simulink model "ST_ESP_ESM_2016a"  (R2016a)
settings: Solver=ode1  StartTime=0.0  StopTime=SIM_time  FixedStep=stepsize  RelTol=1e-3
values from neighbouring files (symbols this model uses):
  A = 2.26    [ST_einspur_parameter.m]
  brems_k_max = 25000    [ST_einspur_parameter.m]
  cw = 0.32    [ST_einspur_parameter.m]
  delta_lr = 0    [ST_einspur_parameter_dynamik.m]    (also in ST_einspur_parameter_sinus.m = 90; ST_einspur_parameter_sprung.m = 90)
  fah_dkv = 0.6    [ST_einspur_parameter_dynamik.m]    (also in ST_einspur_parameter_sinus.m = 0.2; ST_einspur_parameter_sprung.m)
  fzg_Jz = 3489    [ST_einspur_parameter.m]
  fzg_l = 2.758    [ST_einspur_parameter.m]
  fzg_lh = fzg_l-fzg_lv    (= 1.158)    [ST_einspur_parameter.m]
  fzg_lv = 1.6    [ST_einspur_parameter.m]
  fzg_m = 1700    [ST_einspur_parameter.m]
  fzg_s = 1.7    [ST_einspur_parameter.m]
  g = 9.81    [ST_einspur_parameter.m]
  h_sp = 0.56    [ST_einspur_parameter.m]
  i_diff = 3.5    [ST_einspur_parameter.m]
  i_getr = 4.2    [ST_einspur_parameter.m]
  i_lenk = 18    [ST_einspur_parameter.m]
  init_v0 = 5/3.6    (= 1.38888888889)    [ST_einspur_parameter_dynamik.m]    (also in ST_einspur_parameter_sinus.m = 13.8888888889; ST_einspur_parameter_sprung.m = 11.1111111111)
  len_wahl = 1    [ST_einspur_parameter_dynamik.m]    (also in ST_einspur_parameter_sinus.m = 2; ST_einspur_parameter_sprung.m = 3)
  mue_h = 1.0    (= 1)    [ST_einspur_parameter.m]
  mue_v = 1.0    (= 1)    [ST_einspur_parameter.m]
  omega_max = 630    [ST_einspur_parameter.m]
  p_max = 110000    [ST_einspur_parameter.m]
  rad_r = 0.31    [ST_einspur_parameter.m]
  rho = 1.226    [ST_einspur_parameter.m]
  sin_freq = pi/2    (= 1.57079632679)    [ST_einspur_parameter_dynamik.m]    (also in ST_einspur_parameter_sinus.m = 1.0471975512; ST_einspur_parameter_sprung.m)
  step_time = 1    [ST_einspur_parameter_dynamik.m]    (also in ST_einspur_parameter_sinus.m; ST_einspur_parameter_sprung.m = 3)
  sw_ESP = 1    [ST_einspur_parameter_sinus.m]    (also in ST_einspur_parameter_sprung.m)
libraries: simulink x2
(part 1 of 2)
settings Model: Creator=os.alsaidi  LastModifiedBy=Yuheng_Wu
settings DataIOCC: LimitDataPoints=on  SaveFormat=Array
settings HardwareCC: ProdBitPerPointer=32  ProdLargestAtomicFloat=None  ProdIntDivRoundTo=Undefined  ProdEndianess=Unspecified  ProdWordSize=32  ProdHWDeviceType=32-bit Generic
settings ModelReferenceCC: PropagateSignalLabelsOutOfModel=off

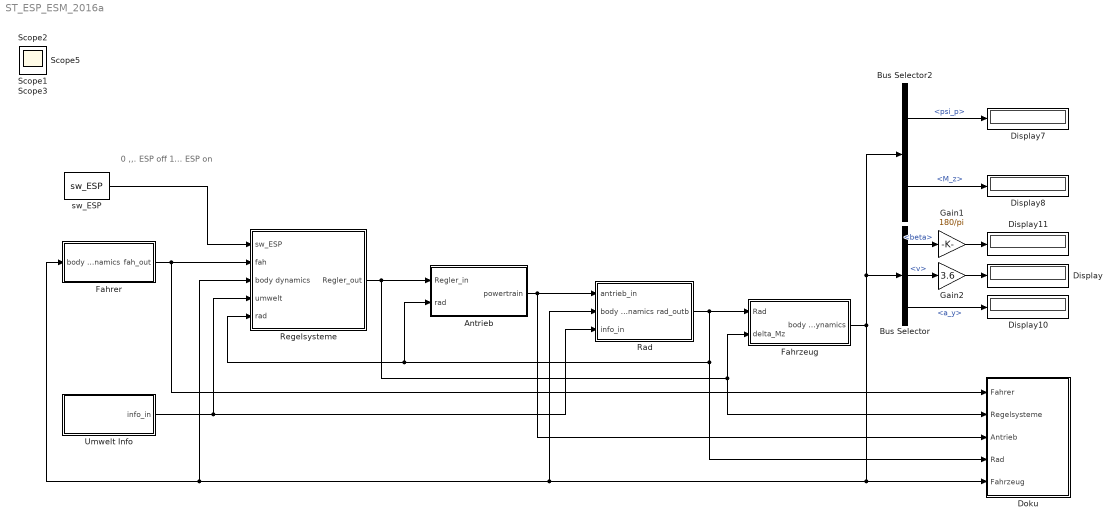
== system ST_ESP_ESM_2016a ==
  note: 0 ,,. ESP off
      | 1... ESP on
  Antrieb : Subsystem
  Bus Selector : BusSelector  OutputSignals=beta,v,a_y
  Bus Selector2 : BusSelector  OutputSignals=psi_p,M_z
  Display{,7..8,10..11} (5 alike) : Display
  Doku : Subsystem
  Fahrer : Subsystem
  Fahrzeug : Subsystem
  Gain1 : Gain  Gain=180/pi
  Gain2 : Gain  Gain=3.6
  Rad : Subsystem
      mask help: Simulink:masks:GenSFuncDesc_MD
      mask Help: eval('feval(''rtwprivate'',''rtwhelpview'',''rtw_sfcn_block'')');
  Regelsysteme : Subsystem
  Umwelt Info : Subsystem
  sw_ESP : Constant  Value=sw_ESP
  Scope{1..3,5} (4 alike) : Scope
  wires:
  Fahrzeug/1(body dynamics) -> Doku/5(Fahrzeug), Rad/2(body dynamics), Regelsysteme/3(body dynamics), Fahrer/1(body dynamics), Bus Selector/1, Bus Selector2/1
  Fahrer/1(fah_out) -> Doku/1(Fahrer), Regelsysteme/2(fah)
  Rad/1(rad_outb) -> Doku/4(Rad), Antrieb/2(rad), Regelsysteme/5(rad), Fahrzeug/1(Rad)
  Antrieb/1(powertrain) -> Rad/1(antrieb_in), Doku/3(Antrieb)
  Bus Selector/2 -> Gain2/1  "<v>"
  Umwelt Info/1(info_in) -> Rad/3(info_in), Regelsysteme/4(umwelt)
  Regelsysteme/1(Regler_out) -> Antrieb/1(Regler_in), Fahrzeug/2(delta_Mz), Doku/2(Regelsysteme)
  Bus Selector/3 -> Display10/1  "<a_y>"
  Bus Selector/1 -> Gain1/1  "<beta>"
  Gain1/1 -> Display11/1
  Gain2/1 -> Display/1
  Bus Selector2/1 -> Display7/1  "<psi_p>"
  Bus Selector2/2 -> Display8/1  "<M_z>"
  sw_ESP/1 -> Regelsysteme/1(sw_ESP)

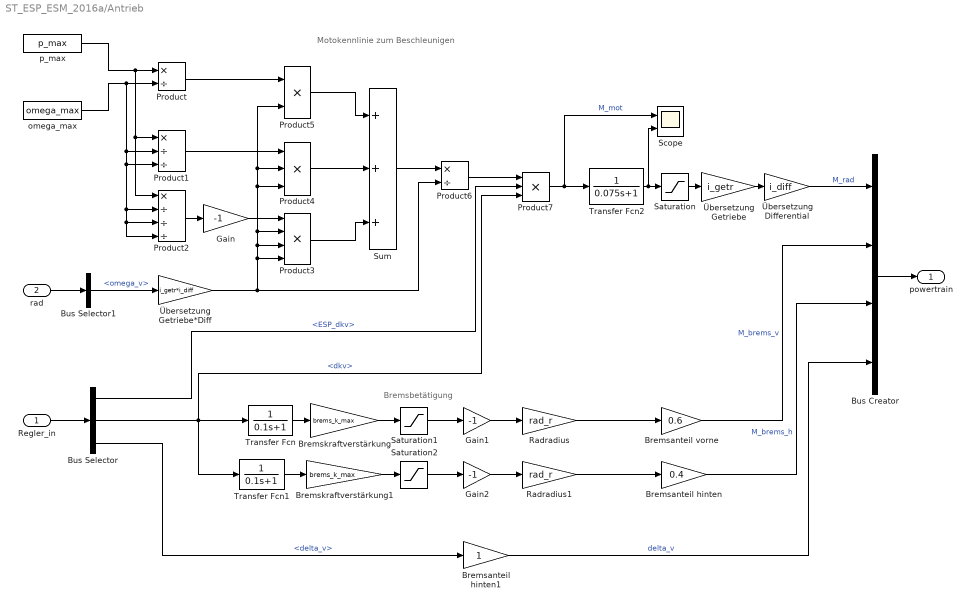
== system ST_ESP_ESM_2016a/Antrieb ==
  note: Motokennlinie zum Beschleunigen
  note: Bremsbetätigung
  Regler_in : Inport
  rad : Inport  Port=2
  Bremsanteil hinten : Gain  Gain=0.4
  Bremsanteil hinten1 : Gain
  Bremsanteil vorne : Gain  Gain=0.6
  Bremskraftverstärkung : Gain  Gain=brems_k_max
  Bremskraftverstärkung1 : Gain  Gain=brems_k_max
  Bus Creator : BusCreator  Inputs=4
  Bus Selector : BusSelector  OutputSignals=ESP.ESP_dkv,fahrer.dkv,fahrer.delta_v
  Bus Selector1 : BusSelector  OutputSignals=omega_v
  Gain : Gain  Gain=-1
  Gain1 : Gain  Gain=-1
  Gain2 : Gain  Gain=-1
  Product : Product  Inputs=*/  RndMeth=Zero
  Product1 : Product  Inputs=*//  RndMeth=Zero
  Product2 : Product  Inputs=*///  RndMeth=Zero
  Product3 : Product  Inputs=4  RndMeth=Zero
  Product4 : Product  Inputs=3  RndMeth=Zero
  Product5 : Product  RndMeth=Zero
  Product6 : Product  Inputs=*/  RndMeth=Zero
  Product7 : Product  Inputs=3  RndMeth=Zero
  Radradius : Gain  Gain=rad_r
  Radradius1 : Gain  Gain=rad_r
  Saturation : Saturate  UpperLimit=inf  LowerLimit=0
  Saturation1 : Saturate  UpperLimit=0  LowerLimit=-inf
  Saturation2 : Saturate  UpperLimit=0  LowerLimit=-inf
  Scope : Scope  NumInputPorts=2
  Sum : Sum  Inputs=+++
  Transfer Fcn : TransferFcn  Denominator=[0.1 1]
  Transfer Fcn1 : TransferFcn  Denominator=[0.1 1]
  Transfer Fcn2 : TransferFcn  Denominator=[0.075 1]
  omega_max : Constant  Value=omega_max
  p_max : Constant  Value=p_max
  Übersetzung Differential : Gain  Gain=i_diff
  Übersetzung Getriebe : Gain  Gain=i_getr
  Übersetzung Getriebe*Diff : Gain  Gain=i_getr*i_diff
  powertrain : Outport
  wires:
  rad/1 -> Bus Selector1/1
  Bus Selector1/1 -> Übersetzung Getriebe*Diff/1  "<omega_v>"
  p_max/1 -> Product/1, Product1/1, Product2/1
  omega_max/1 -> Product/2, Product1/2, Product1/3, Product2/2, Product2/3, Product2/4
  Product/1 -> Product5/1
  Product2/1 -> Gain/1
  Product1/1 -> Product4/1
  Gain/1 -> Product3/1
  Product5/1 -> Sum/1
  Product4/1 -> Sum/2
  Product3/1 -> Sum/3
  Sum/1 -> Product6/1
  Product6/1 -> Product7/1
  Product7/1 -> Scope/1, Transfer Fcn2/1  "M_mot"
  Übersetzung Getriebe/1 -> Übersetzung Differential/1
  Übersetzung Differential/1 -> Bus Creator/1  "M_rad"
  Bus Creator/1 -> powertrain/1
  Saturation/1 -> Übersetzung Getriebe/1
  Bremskraftverstärkung/1 -> Saturation1/1
  Saturation1/1 -> Gain1/1
  Gain1/1 -> Radradius/1
  Bremsanteil vorne/1 -> Bus Creator/2  "M_brems_v"
  Radradius/1 -> Bremsanteil vorne/1
  Bremsanteil hinten/1 -> Bus Creator/3  "M_brems_h"
  Bremskraftverstärkung1/1 -> Saturation2/1
  Saturation2/1 -> Gain2/1
  Gain2/1 -> Radradius1/1
  Radradius1/1 -> Bremsanteil hinten/1
  Regler_in/1 -> Bus Selector/1
  Bus Selector/3 -> Bremsanteil hinten1/1  "<delta_v>"
  Bus Selector/2 -> Product7/3, Transfer Fcn/1, Transfer Fcn1/1  "<dkv>"
  Übersetzung Getriebe*Diff/1 -> Product3/3, Product3/2, Product4/3, Product4/2, Product5/2, Product3/4, Product6/2
  Transfer Fcn/1 -> Bremskraftverstärkung/1
  Transfer Fcn1/1 -> Bremskraftverstärkung1/1
  Transfer Fcn2/1 -> Scope/2, Saturation/1
  Bremsanteil hinten1/1 -> Bus Creator/4  "delta_v"
  Bus Selector/1 -> Product7/2  "<ESP_dkv>"

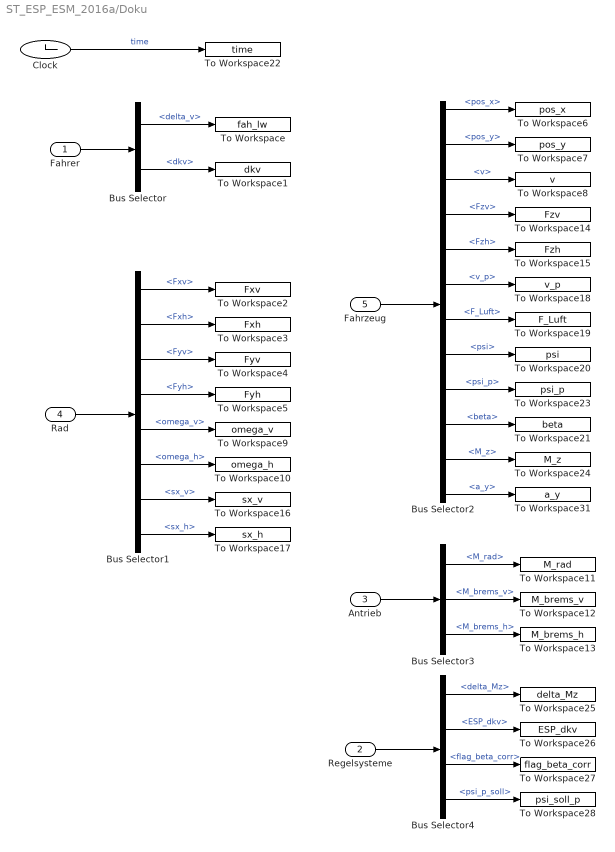
== system ST_ESP_ESM_2016a/Doku ==
  Fahrer : Inport
  Regelsysteme : Inport  Port=2
  Antrieb : Inport  Port=3
  Rad : Inport  Port=4
  Fahrzeug : Inport  Port=5
  Bus Selector : BusSelector  OutputSignals=delta_v,dkv
  Bus Selector1 : BusSelector  OutputSignals=Fxv,Fxh,Fyv,Fyh,omega_v,omega_h,sx_v,sx_h
  Bus Selector2 : BusSelector  OutputSignals=pos_x,pos_y,v,Fzv,Fzh,v_p,F_Luft,psi,psi_p,beta,M_z,a_y
  Bus Selector3 : BusSelector  OutputSignals=M_rad,M_brems_v,M_brems_h
  Bus Selector4 : BusSelector  OutputSignals=ESP.delta_Mz,ESP.ESP_dkv,ESP.flag_beta_corr,ESP.psi_p_soll
  Clock : Clock
  To Workspace : ToWorkspace  VariableName=fah_lw  SampleTime=-1
  To Workspace1 : ToWorkspace  VariableName=dkv  SampleTime=-1
  To Workspace10 : ToWorkspace  VariableName=omega_h  SampleTime=-1
  To Workspace11 : ToWorkspace  VariableName=M_rad  SampleTime=-1
  To Workspace12 : ToWorkspace  VariableName=M_brems_v  SampleTime=-1
  To Workspace13 : ToWorkspace  VariableName=M_brems_h  SampleTime=-1
  To Workspace14 : ToWorkspace  VariableName=Fzv  SampleTime=-1
  To Workspace15 : ToWorkspace  VariableName=Fzh  SampleTime=-1
  To Workspace16 : ToWorkspace  VariableName=sx_v  SampleTime=-1
  To Workspace17 : ToWorkspace  VariableName=sx_h  SampleTime=-1
  To Workspace18 : ToWorkspace  VariableName=v_p  SampleTime=-1
  To Workspace19 : ToWorkspace  VariableName=F_Luft  SampleTime=-1
  To Workspace2 : ToWorkspace  VariableName=Fxv  SampleTime=-1
  To Workspace20 : ToWorkspace  VariableName=psi  SampleTime=-1
  To Workspace21 : ToWorkspace  VariableName=beta  SampleTime=-1
  To Workspace22 : ToWorkspace  VariableName=time  SampleTime=-1
  To Workspace23 : ToWorkspace  VariableName=psi_p  SampleTime=-1
  To Workspace24 : ToWorkspace  VariableName=M_z  SampleTime=-1
  To Workspace25 : ToWorkspace  VariableName=delta_Mz  SampleTime=-1
  To Workspace26 : ToWorkspace  VariableName=ESP_dkv  SampleTime=-1
  To Workspace27 : ToWorkspace  VariableName=flag_beta_corr  SampleTime=-1
  To Workspace28 : ToWorkspace  VariableName=psi_soll_p  SampleTime=-1
      settings: Save2DSignal=2-D array (concatenate along first dimension)
  To Workspace3 : ToWorkspace  VariableName=Fxh  SampleTime=-1
  To Workspace31 : ToWorkspace  VariableName=a_y  SampleTime=-1
  To Workspace4 : ToWorkspace  VariableName=Fyv  SampleTime=-1
  To Workspace5 : ToWorkspace  VariableName=Fyh  SampleTime=-1
  To Workspace6 : ToWorkspace  VariableName=pos_x  SampleTime=-1
  To Workspace7 : ToWorkspace  VariableName=pos_y  SampleTime=-1
  To Workspace8 : ToWorkspace  VariableName=v  SampleTime=-1
  To Workspace9 : ToWorkspace  VariableName=omega_v  SampleTime=-1
  wires:
  Fahrer/1 -> Bus Selector/1
  Rad/1 -> Bus Selector1/1
  Fahrzeug/1 -> Bus Selector2/1
  Bus Selector/1 -> To Workspace/1  "<delta_v>"
  Bus Selector/2 -> To Workspace1/1  "<dkv>"
  Bus Selector1/1 -> To Workspace2/1  "<Fxv>"
  Bus Selector1/2 -> To Workspace3/1  "<Fxh>"
  Bus Selector1/3 -> To Workspace4/1  "<Fyv>"
  Bus Selector1/4 -> To Workspace5/1  "<Fyh>"
  Bus Selector2/1 -> To Workspace6/1  "<pos_x>"
  Bus Selector2/2 -> To Workspace7/1  "<pos_y>"
  Bus Selector2/3 -> To Workspace8/1  "<v>"
  Regelsysteme/1 -> Bus Selector4/1
  Bus Selector1/5 -> To Workspace9/1  "<omega_v>"
  Bus Selector1/6 -> To Workspace10/1  "<omega_h>"
  Antrieb/1 -> Bus Selector3/1
  Bus Selector3/1 -> To Workspace11/1  "<M_rad>"
  Bus Selector3/2 -> To Workspace12/1  "<M_brems_v>"
  Bus Selector3/3 -> To Workspace13/1  "<M_brems_h>"
  Bus Selector2/4 -> To Workspace14/1  "<Fzv>"
  Bus Selector2/5 -> To Workspace15/1  "<Fzh>"
  Bus Selector1/7 -> To Workspace16/1  "<sx_v>"
  Bus Selector1/8 -> To Workspace17/1  "<sx_h>"
  Bus Selector2/6 -> To Workspace18/1  "<v_p>"
  Bus Selector2/7 -> To Workspace19/1  "<F_Luft>"
  Bus Selector2/8 -> To Workspace20/1  "<psi>"
  Bus Selector2/10 -> To Workspace21/1  "<beta>"
  Clock/1 -> To Workspace22/1  "time"
  Bus Selector2/9 -> To Workspace23/1  "<psi_p>"
  Bus Selector2/11 -> To Workspace24/1  "<M_z>"
  Bus Selector4/1 -> To Workspace25/1  "<delta_Mz>"
  Bus Selector2/12 -> To Workspace31/1  "<a_y>"
  Bus Selector4/2 -> To Workspace26/1  "<ESP_dkv>"
  Bus Selector4/3 -> To Workspace27/1  "<flag_beta_corr>"
  Bus Selector4/4 -> To Workspace28/1  "<psi_p_soll>"

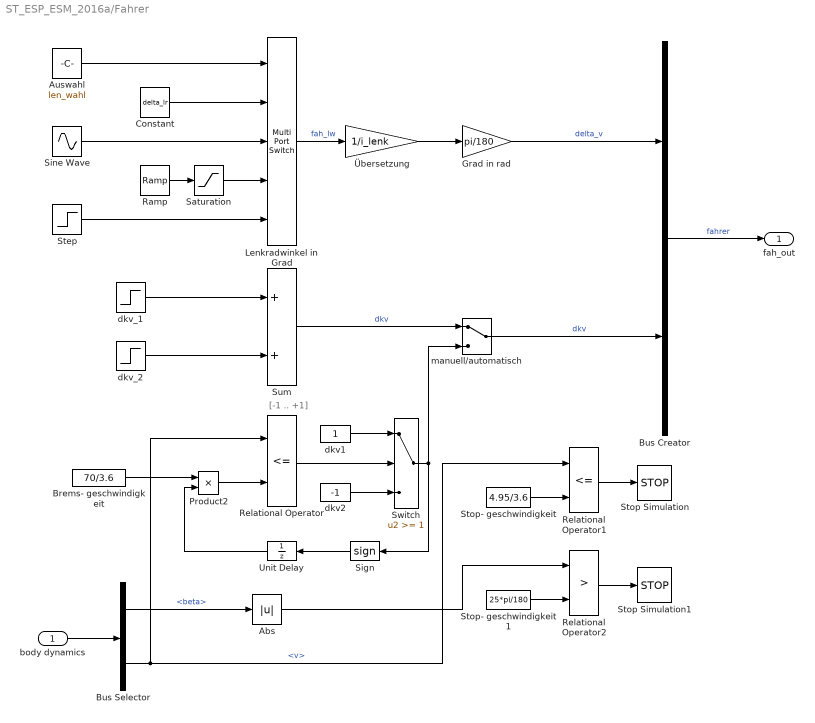
== system ST_ESP_ESM_2016a/Fahrer ==
  note: [-1 .. +1]
  body dynamics : Inport
  Abs : Abs
  Auswahl : Constant  Value=len_wahl
  Brems- geschwindigkeit : Constant  Value=70/3.6
  Bus Creator : BusCreator  Inputs=2
  Bus Selector : BusSelector  OutputSignals=beta,v
  Constant : Constant  Value=delta_lr
  Grad in rad : Gain  Gain=pi/180
  Lenkradwinkel in Grad : MultiPortSwitch  Inputs=4
  Product2 : Product  RndMeth=Zero
  Ramp : simulink/Sources/Ramp  slope=180/pi  start=step_time  X0=0
  Relational Operator : RelationalOperator  Operator=<=  OutDataTypeStr=boolean
  Relational Operator1 : RelationalOperator  Operator=<=  OutDataTypeStr=boolean
  Relational Operator2 : RelationalOperator  Operator=>  OutDataTypeStr=boolean
  Saturation : Saturate  UpperLimit=delta_lr  LowerLimit=-delta_lr
  Sign : Signum
  Sine Wave : Sin  Amplitude=delta_lr  Frequency=sin_freq  SampleTime=0
  Step : Step  Time=step_time+3  After=delta_lr  SampleTime=0
  Stop Simulation : Stop
  Stop Simulation1 : Stop
  Stop- geschwindigkeit : Constant  Value=4.95/3.6
  Stop- geschwindigkeit1 : Constant  Value=25*pi/180
  Sum : Sum
  Switch : Switch  Threshold=1
  Unit Delay : UnitDelay  InitialCondition=1  SampleTime=-1
  dkv1 : Constant
  dkv2 : Constant  Value=-1
  dkv_1 : Step  Time=0  Before=fah_dkv  After=fah_dkv  SampleTime=0
  dkv_2 : Step  Time=0  After=0  SampleTime=0
  manuell/automatisch : ManualSwitch
  Übersetzung : Gain  Gain=1/i_lenk
  fah_out : Outport
  wires:
  Auswahl/1 -> Lenkradwinkel in Grad/1
  Constant/1 -> Lenkradwinkel in Grad/2
  Sine Wave/1 -> Lenkradwinkel in Grad/3
  Ramp/1 -> Saturation/1
  Saturation/1 -> Lenkradwinkel in Grad/4
  dkv_1/1 -> Sum/1
  dkv_2/1 -> Sum/2
  Lenkradwinkel in Grad/1 -> Übersetzung/1  "fah_lw"
  Bus Creator/1 -> fah_out/1  "fahrer"
  Grad in rad/1 -> Bus Creator/1  "delta_v"
  manuell/automatisch/1 -> Bus Creator/2  "dkv"
  Sum/1 -> manuell/automatisch/1  "dkv"
  Relational Operator/1 -> Switch/2
  Switch/1 -> manuell/automatisch/2, Sign/1
  dkv1/1 -> Switch/1
  dkv2/1 -> Switch/3
  Brems- geschwindigkeit/1 -> Product2/1
  Product2/1 -> Relational Operator/2
  Unit Delay/1 -> Product2/2
  Sign/1 -> Unit Delay/1
  Stop- geschwindigkeit/1 -> Relational Operator1/2
  Relational Operator1/1 -> Stop Simulation/1
  Step/1 -> Lenkradwinkel in Grad/5
  Stop- geschwindigkeit1/1 -> Relational Operator2/2
  Relational Operator2/1 -> Stop Simulation1/1
  Übersetzung/1 -> Grad in rad/1
  body dynamics/1 -> Bus Selector/1
  Bus Selector/2 -> Relational Operator/1, Relational Operator1/1  "<v>"
  Bus Selector/1 -> Abs/1  "<beta>"
  Abs/1 -> Relational Operator2/1

== system ST_ESP_ESM_2016a/Fahrzeug ==
  Rad : Inport
  delta_Mz : Inport  Port=2
  "Bewegungsgleichungen " : Subsystem
  Bus Creator : BusCreator  Inputs=18
  Bus Selector : BusSelector  OutputSignals=Fxv,Fxh,Fyv,Fyh,delta_v
  Bus Selector2 : BusSelector  OutputSignals=ESP.delta_Mz
  Memory : Memory  X0=fzg_m*g*fzg_lh/(fzg_lh+fzg_lv)
  Memory1 : Memory  X0=fzg_m*g*fzg_lv/(fzg_lh+fzg_lv)
  Radaufstandskräfte : Subsystem
  x-y-Koordinaten : Subsystem
  body dynamics : Outport
  wires:
  Bus Selector2/1 -> "Bewegungsgleichungen "/6(delta_Mz)  "<delta_Mz>"
  delta_Mz/1 -> Bus Selector2/1
  "Bewegungsgleichungen "/9(a_x) -> Radaufstandskräfte/1(a_x), Bus Creator/16  "a_x"
  "Bewegungsgleichungen "/1(psi) -> Bus Creator/8, x-y-Koordinaten/1(psi)
  "Bewegungsgleichungen "/3(v) -> Bus Creator/10, x-y-Koordinaten/3(v)
  x-y-Koordinaten/2(pos_y) -> Bus Creator/7  "pos_y"
  Bus Selector/1 -> Bus Creator/1, "Bewegungsgleichungen "/1(Fxv)  "<Fxv>"
  Bus Selector/2 -> Bus Creator/2, "Bewegungsgleichungen "/2(Fxh)  "<Fxh>"
  Bus Selector/3 -> Bus Creator/3, "Bewegungsgleichungen "/3(Fyv)  "<Fyv>"
  Bus Selector/4 -> Bus Creator/4, "Bewegungsgleichungen "/4(Fyh)  "<Fyh>"
  Bus Selector/5 -> Bus Creator/5, "Bewegungsgleichungen "/5(delta_v)  "<delta_v>"
  Rad/1 -> Bus Selector/1
  Bus Creator/1 -> body dynamics/1
  x-y-Koordinaten/1(pos_x) -> Bus Creator/6  "pos_x"
  "Bewegungsgleichungen "/5(F_Luft) -> Radaufstandskräfte/2(F_luft), Bus Creator/12
  "Bewegungsgleichungen "/6(psi_p) -> Bus Creator/13
  Memory1/1 -> Bus Creator/18  "Fzh"
  Memory/1 -> Bus Creator/17  "Fzv"
  "Bewegungsgleichungen "/7(a_y) -> Bus Creator/14  "a_y"
  "Bewegungsgleichungen "/8(M_z) -> Bus Creator/15  "M_z"
  "Bewegungsgleichungen "/2(beta) -> Bus Creator/9, x-y-Koordinaten/2(beta)
  Radaufstandskräfte/1(Fzv) -> Memory/1
  Radaufstandskräfte/2(Fzh) -> Memory1/1
  "Bewegungsgleichungen "/4(v_p) -> Bus Creator/11  "v_p"

== system ST_ESP_ESM_2016a/Rad ==
  antrieb_in : Inport
  body dynamics : Inport  Port=2
  info_in : Inport  Port=3
  Rad_sfcn : S-Function  FunctionName=Rad_sf  SFunctionModules=""  SFunctionDeploymentMode=off  EnableBusSupport=off  mask{rtw_sf_name=Rad_sf, showVar=off}
      mask prompts: rtw_sf_name "Simulink:masks:GenSFuncName_MP"; showVar "Simulink:masks:GenSFuncShowModuleList_MP"
      mask help: Simulink:masks:GenSFuncDesc_MD
      mask init:
      | displist = '';
      | if ~strcmp(get_param(gcb, 'FunctionName'), rtw_sf_name);
      |   set_param(gcb, 'FunctionName', rtw_sf_name);
      | end
      | % Check if we are generating code
      | rtw_mode = false;
      | if strcmpi(get_param(bdroot(gcb),'SimulationStatus'),'Initializing')
      | 	rtw_mode = strcmpi(get_param(bdroot(gcb),'BuildingRTWCode'),'on') && ...
      | 		~strcmpi(get_param(bdroot(gcb),'TargetStyle'),'SimulationTarget');
      | end
      | if showVar || rtw_mode
      | 	if exist('rtwsfunc') == 2 | exist('rtwsfunc') == 6
      | 		tmplist = rtwsfunc(rtw_sf_name,gcb);
      | 		tmplist = DAStudio.message('Simulink:masks:GenSFuncListOfModules_IC', tmplist);
      | 	elseif showVar
      | 		tmplist1 = DAStudio.message('Simulink:masks:GenSFuncListOfModules_IC', '');
      |         tmplist2 = DAStudio.message('Simulink:masks:GenSFuncNotLicensed_IC');
      |         tmplist = [tmplist1 tmplist2];
      |  	end
      | end
      | if showVar
      |   displist = tmplist;
      | end
      settings: CopyFcn=|
      | if ~strcmp(get_param(gcb,'Linkstatus'),'none') && ...
      | ~strcmp(get_param(gcb,'Linkstatus'),'implicit')
      |   set_param(gcb,'LinkStatus','none');
      | end
      mask Help: eval('feval(''rtwprivate'',''rtwhelpview'',''rtw_sfcn_block'')');
      mask Display:
      | port_label('input',1,'M_rad');
      | port_label('input',2,'M_brems_v');
      | port_label('input',3,'M_brems_h');
      | port_label('input',4,'delta_v');
      | port_label('input',5,'Fxv');
      | port_label('input',6,'Fxh');
      | port_label('input',7,'Fyv');
      | port_label('input',8,'Fyh');
      | port_label('input',9,'delta_vb');
      | port_label('input',10,'pos_x');
      | port_label('input',11,'pos_y');
      | port_label('input',12,'psi');
      | port_label('input',13,'beta');
      | port_label('input',14,'v');
      | port_label('input',15,'v_p');
      | port_label('input',16,'F_Luft');
      | port_label('input',17,'psi_p');
      | port_label('input',18,'a_y');
      | port_label('input',19,'M_z');
      | port_label('input',20,'a_x');
      | port_label('input',21,'Fzv');
      | port_label('input',22,'Fzh');
      | port_label('input',23,'rad_mue_vl');
      | port_label('input',24,'rad_mue_hl');
      | port_label('output',1,'Fxvb');
      | port_label('output',2,'Fyvb');
      | port_label('output',3,'Fxhb');
      | port_label('output',4,'Fyhb');
      | port_label('output',5,'delta_va');
      | port_label('output',6,'scaling_fkt_v');
      | port_label('output',7,'scaling_fkt_h');
      | port_label('output',8,'sx_v');
      | port_label('output',9,'sx_h');
      | port_label('output',10,'omega_h');
      | port_label('output',11,'omega_v');
      | port_label('output',12,'sx_flag_v');
      | port_label('output',13,'sx_flag_h');
      | port_label('output',14,'sy_v');
      | port_label('output',15,'sy_h');
      | port_label('output',16,'rad_n_ges_v');
      | port_label('output',17,'rad_M_z_v');
      | port_label('output',18,'rad_n_ges_h');
      | port_label('output',19,'rad_M_z_h');
      | port_label('output',20,'s_abs_v');
      | port_label('output',21,'s_abs_h');
  __InputSSForSFun__ : Subsystem
      settings: PermitHierarchicalResolution=ParametersOnly
  __OutputSSForSFun__ : Subsystem
      settings: PermitHierarchicalResolution=ParametersOnly
  rad_outb : Outport
  wires:
  __OutputSSForSFun__/1(rad_outb) -> rad_outb/1
  Rad_sfcn/21 -> __OutputSSForSFun__/21(__UniqueInportName__21__)
  Rad_sfcn/20 -> __OutputSSForSFun__/20(__UniqueInportName__20__)
  Rad_sfcn/19 -> __OutputSSForSFun__/19(__UniqueInportName__19__)
  Rad_sfcn/18 -> __OutputSSForSFun__/18(__UniqueInportName__18__)
  Rad_sfcn/17 -> __OutputSSForSFun__/17(__UniqueInportName__17__)
  Rad_sfcn/16 -> __OutputSSForSFun__/16(__UniqueInportName__16__)
  Rad_sfcn/15 -> __OutputSSForSFun__/15(__UniqueInportName__15__)
  Rad_sfcn/14 -> __OutputSSForSFun__/14(__UniqueInportName__14__)
  Rad_sfcn/13 -> __OutputSSForSFun__/13(__UniqueInportName__13__)
  Rad_sfcn/12 -> __OutputSSForSFun__/12(__UniqueInportName__12__)
  Rad_sfcn/11 -> __OutputSSForSFun__/11(__UniqueInportName__11__)
  Rad_sfcn/10 -> __OutputSSForSFun__/10(__UniqueInportName__10__)
  Rad_sfcn/9 -> __OutputSSForSFun__/9(__UniqueInportName__9__)
  Rad_sfcn/8 -> __OutputSSForSFun__/8(__UniqueInportName__8__)
  Rad_sfcn/7 -> __OutputSSForSFun__/7(__UniqueInportName__7__)
  Rad_sfcn/6 -> __OutputSSForSFun__/6(__UniqueInportName__6__)
  Rad_sfcn/5 -> __OutputSSForSFun__/5(__UniqueInportName__5__)
  Rad_sfcn/4 -> __OutputSSForSFun__/4(__UniqueInportName__4__)
  Rad_sfcn/3 -> __OutputSSForSFun__/3(__UniqueInportName__3__)
  Rad_sfcn/2 -> __OutputSSForSFun__/2(__UniqueInportName__2__)
  Rad_sfcn/1 -> __OutputSSForSFun__/1(__UniqueInportName__1__)
  __InputSSForSFun__/24(__UniqueOutportName__24__) -> Rad_sfcn/24
  __InputSSForSFun__/23(__UniqueOutportName__23__) -> Rad_sfcn/23
  __InputSSForSFun__/22(__UniqueOutportName__22__) -> Rad_sfcn/22
  __InputSSForSFun__/21(__UniqueOutportName__21__) -> Rad_sfcn/21
  __InputSSForSFun__/20(__UniqueOutportName__20__) -> Rad_sfcn/20
  __InputSSForSFun__/19(__UniqueOutportName__19__) -> Rad_sfcn/19
  __InputSSForSFun__/18(__UniqueOutportName__18__) -> Rad_sfcn/18
  __InputSSForSFun__/17(__UniqueOutportName__17__) -> Rad_sfcn/17
  __InputSSForSFun__/16(__UniqueOutportName__16__) -> Rad_sfcn/16
  __InputSSForSFun__/15(__UniqueOutportName__15__) -> Rad_sfcn/15
  __InputSSForSFun__/14(__UniqueOutportName__14__) -> Rad_sfcn/14
  __InputSSForSFun__/13(__UniqueOutportName__13__) -> Rad_sfcn/13
  __InputSSForSFun__/12(__UniqueOutportName__12__) -> Rad_sfcn/12
  __InputSSForSFun__/11(__UniqueOutportName__11__) -> Rad_sfcn/11
  __InputSSForSFun__/10(__UniqueOutportName__10__) -> Rad_sfcn/10
  __InputSSForSFun__/9(__UniqueOutportName__9__) -> Rad_sfcn/9
  __InputSSForSFun__/8(__UniqueOutportName__8__) -> Rad_sfcn/8
  __InputSSForSFun__/7(__UniqueOutportName__7__) -> Rad_sfcn/7
  __InputSSForSFun__/6(__UniqueOutportName__6__) -> Rad_sfcn/6
  __InputSSForSFun__/5(__UniqueOutportName__5__) -> Rad_sfcn/5
  __InputSSForSFun__/4(__UniqueOutportName__4__) -> Rad_sfcn/4
  __InputSSForSFun__/3(__UniqueOutportName__3__) -> Rad_sfcn/3
  __InputSSForSFun__/2(__UniqueOutportName__2__) -> Rad_sfcn/2
  __InputSSForSFun__/1(__UniqueOutportName__1__) -> Rad_sfcn/1
  info_in/1 -> __InputSSForSFun__/3(info_in)
  body dynamics/1 -> __InputSSForSFun__/2(body dynamics)
  antrieb_in/1 -> __InputSSForSFun__/1(antrieb_in)

== system ST_ESP_ESM_2016a/Regelsysteme ==
  sw_ESP : Inport
  fah : Inport  Port=2
  body dynamics : Inport  Port=3
  umwelt : Inport  Port=4
  rad : Inport  Port=5
  Bus Creator1 : BusCreator  Inputs=2
  Bus Creator2 : BusCreator  Inputs=4
  ESP : Subsystem
  Gain{1..4} (4 alike) : Gain
  Product : Product  RndMeth=Zero
  Regler_out : Outport
  wires:
  fah/1 -> Bus Creator1/2, ESP/4(fah)
  rad/1 -> ESP/2(Rad)
  Bus Creator1/1 -> Regler_out/1  "regler_out"
  ESP/1(delta_Mz) -> Product/2
  body dynamics/1 -> ESP/1(body dynamics)
  umwelt/1 -> ESP/3(umwelt)
  Bus Creator2/1 -> Bus Creator1/1  "ESP"
  Product/1 -> Gain4/1
  ESP/2(ESP_dkv) -> Gain3/1
  ESP/3(flag_beta_corr) -> Gain2/1
  sw_ESP/1 -> Product/1
  ESP/4(psi_p_soll) -> Gain1/1
  Gain1/1 -> Bus Creator2/4  "psi_p_soll"
  Gain2/1 -> Bus Creator2/3  "flag_beta_corr"
  Gain3/1 -> Bus Creator2/2  "ESP_dkv"
  Gain4/1 -> Bus Creator2/1  "delta_Mz"

== system ST_ESP_ESM_2016a/Umwelt Info ==
  Bus Creator : BusCreator  Inputs=1
  mue_konst : Subsystem
  info_in : Outport
  wires:
  Bus Creator/1 -> info_in/1  "rad_mue"
  mue_konst/1(rad_mue) -> Bus Creator/1

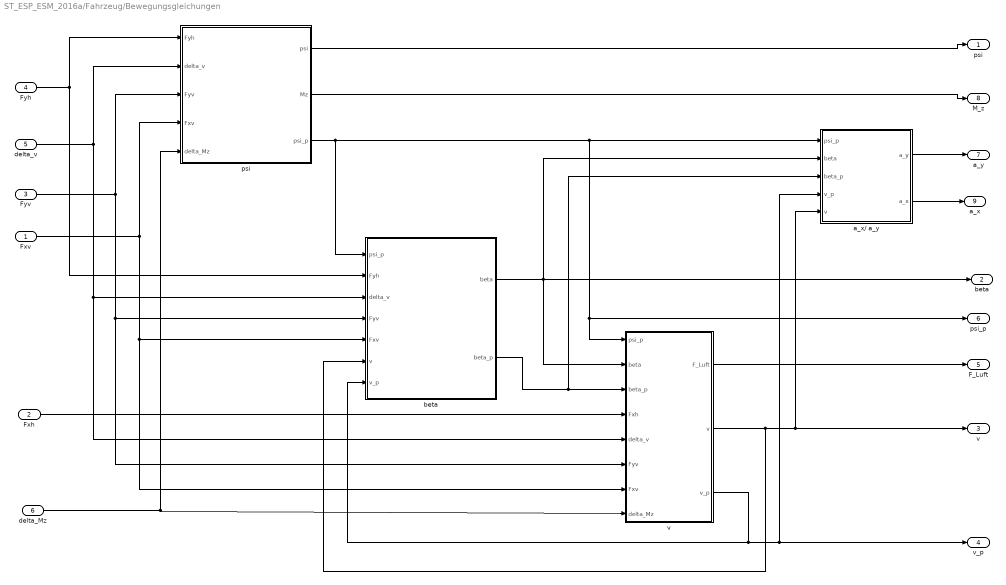
== system ST_ESP_ESM_2016a/Fahrzeug/Bewegungsgleichungen  ==
  Fxv : Inport
  Fxh : Inport  Port=2
  Fyv : Inport  Port=3
  Fyh : Inport  Port=4
  delta_v : Inport  Port=5
  delta_Mz : Inport  Port=6
  a_x/ a_y : Subsystem
  "beta " : Subsystem
  "psi " : Subsystem
  "v " : Subsystem
  psi : Outport
  beta : Outport  Port=2
  v : Outport  Port=3
  v_p : Outport  Port=4
  F_Luft : Outport  Port=5
  psi_p : Outport  Port=6
  a_y : Outport  Port=7
  M_z : Outport  Port=8
  a_x : Outport  Port=9
  wires:
  delta_Mz/1 -> "v "/8(delta_Mz), "psi "/5(delta_Mz)
  delta_v/1 -> "psi "/2(delta_v), "v "/5(delta_v), "beta "/3(delta_v)
  Fyv/1 -> "v "/6(Fyv), "beta "/4(Fyv), "psi "/3(Fyv)
  Fxv/1 -> "v "/7(Fxv), "beta "/5(Fxv), "psi "/4(Fxv)
  "psi "/1(psi) -> psi/1
  "psi "/3(psi_p) -> a_x/ a_y/1(psi_p), psi_p/1, "v "/1(psi_p), "beta "/1(psi_p)
  Fyh/1 -> "beta "/2(Fyh), "psi "/1(Fyh)
  "beta "/1(beta) -> beta/1, a_x/ a_y/2(beta), "v "/2(beta)
  "beta "/2(beta_p) -> a_x/ a_y/3(beta_p), "v "/3(beta_p)
  "v "/2(v) -> "beta "/6(v), a_x/ a_y/5(v), v/1
  "v "/3(v_p) -> a_x/ a_y/4(v_p), v_p/1, "beta "/7(v_p)
  Fxh/1 -> "v "/4(Fxh)
  "v "/1(F_Luft) -> F_Luft/1
  a_x/ a_y/1(a_y) -> a_y/1
  a_x/ a_y/2(a_x) -> a_x/1
  "psi "/2(Mz) -> M_z/1

== system ST_ESP_ESM_2016a/Fahrzeug/Radaufstandskräfte ==
  a_x : Inport
  F_luft : Inport  Port=2
  Add : Sum
  Add1 : Sum  Inputs=+-
  Add2 : Sum
  Constant : Constant  Value=fzg_m
  Gain : Gain  Gain=h_sp/fzg_l
  Gain1 : Gain  Gain=fzg_lv/fzg_l*g
  Gain3 : Gain  Gain=fzg_lh/fzg_l*g
  Product : Product
  Saturation : Saturate  UpperLimit=fzg_m*g  LowerLimit=0
  Saturation1 : Saturate  UpperLimit=fzg_m*g  LowerLimit=0
  Fzv : Outport
  Fzh : Outport  Port=2
  wires:
  a_x/1 -> Product/2
  F_luft/1 -> Add2/2
  Add/1 -> Saturation/1
  Add1/1 -> Saturation1/1
  Constant/1 -> Gain1/1, Product/1, Gain3/1
  Gain/1 -> Add/2, Add1/2
  Gain3/1 -> Add1/1  "m_v*g"
  Gain1/1 -> Add/1  "m_h*g"
  Saturation/1 -> Fzh/1
  Saturation1/1 -> Fzv/1
  Add2/1 -> Gain/1
  Product/1 -> Add2/1

== system ST_ESP_ESM_2016a/Fahrzeug/x-y-Koordinaten ==
  psi : Inport
  beta : Inport  Port=2
  v : Inport  Port=3
  Fcn : Fcn  Expr=cos(u)
  Fcn1 : Fcn  Expr=sin(u)
  Integrator : Integrator
  Integrator1 : Integrator
  Product : Product  RndMeth=Zero
  Product1 : Product  RndMeth=Zero
  Sum : Sum
  pos_x : Outport
  pos_y : Outport  Port=2
  wires:
  v/1 -> Product/2, Product1/2
  Fcn/1 -> Product/1
  Product/1 -> Integrator/1  "v_x"
  psi/1 -> Sum/1
  beta/1 -> Sum/2
  Sum/1 -> Fcn/1, Fcn1/1
  Fcn1/1 -> Product1/1
  Product1/1 -> Integrator1/1  "v_y"
  Integrator/1 -> pos_x/1
  Integrator1/1 -> pos_y/1

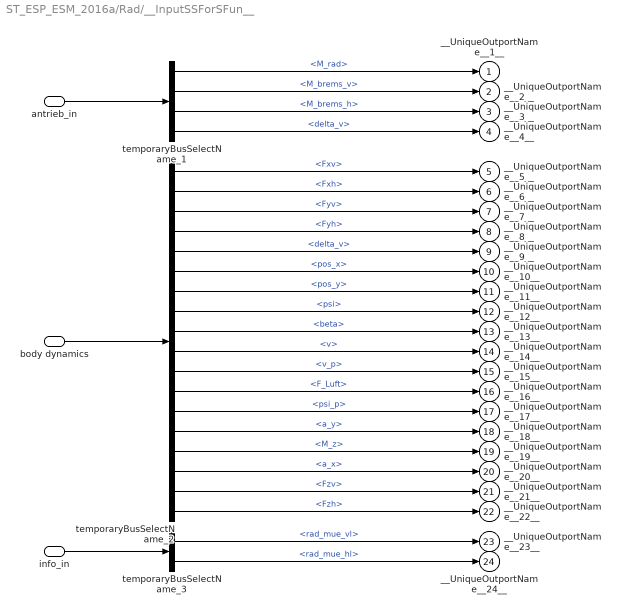
== system ST_ESP_ESM_2016a/Rad/__InputSSForSFun__ ==
  antrieb_in : Inport
  body dynamics : Inport  Port=2
  info_in : Inport  Port=3
  temporaryBusSelectName_1 : BusSelector  OutputSignals=M_rad,M_brems_v,M_brems_h,delta_v
  temporaryBusSelectName_2 : BusSelector  OutputSignals=Fxv,Fxh,Fyv,Fyh,delta_v,pos_x,pos_y,psi,beta,v,v_p,F_Luft,psi_p,a_y,M_z,a_x,Fzv,Fzh
  temporaryBusSelectName_3 : BusSelector  OutputSignals=rad_mue.rad_mue_vl,rad_mue.rad_mue_hl
  __UniqueOutportName__1__ : Outport
  __UniqueOutportName__2__ : Outport  Port=2
  __UniqueOutportName__3__ : Outport  Port=3
  __UniqueOutportName__4__ : Outport  Port=4
  __UniqueOutportName__5__ : Outport  Port=5
  __UniqueOutportName__6__ : Outport  Port=6
  __UniqueOutportName__7__ : Outport  Port=7
  __UniqueOutportName__8__ : Outport  Port=8
  __UniqueOutportName__9__ : Outport  Port=9
  __UniqueOutportName__10__ : Outport  Port=10
  __UniqueOutportName__11__ : Outport  Port=11
  __UniqueOutportName__12__ : Outport  Port=12
  __UniqueOutportName__13__ : Outport  Port=13
  __UniqueOutportName__14__ : Outport  Port=14
  __UniqueOutportName__15__ : Outport  Port=15
  __UniqueOutportName__16__ : Outport  Port=16
  __UniqueOutportName__17__ : Outport  Port=17
  __UniqueOutportName__18__ : Outport  Port=18
  __UniqueOutportName__19__ : Outport  Port=19
  __UniqueOutportName__20__ : Outport  Port=20
  __UniqueOutportName__21__ : Outport  Port=21
  __UniqueOutportName__22__ : Outport  Port=22
  __UniqueOutportName__23__ : Outport  Port=23
  __UniqueOutportName__24__ : Outport  Port=24
  wires:
  temporaryBusSelectName_3/2 -> __UniqueOutportName__24__/1  "<rad_mue_hl>"
  temporaryBusSelectName_3/1 -> __UniqueOutportName__23__/1  "<rad_mue_vl>"
  temporaryBusSelectName_2/18 -> __UniqueOutportName__22__/1  "<Fzh>"
  temporaryBusSelectName_2/17 -> __UniqueOutportName__21__/1  "<Fzv>"
  temporaryBusSelectName_2/16 -> __UniqueOutportName__20__/1  "<a_x>"
  temporaryBusSelectName_2/15 -> __UniqueOutportName__19__/1  "<M_z>"
  temporaryBusSelectName_2/14 -> __UniqueOutportName__18__/1  "<a_y>"
  temporaryBusSelectName_2/13 -> __UniqueOutportName__17__/1  "<psi_p>"
  temporaryBusSelectName_2/12 -> __UniqueOutportName__16__/1  "<F_Luft>"
  temporaryBusSelectName_2/11 -> __UniqueOutportName__15__/1  "<v_p>"
  temporaryBusSelectName_2/10 -> __UniqueOutportName__14__/1  "<v>"
  temporaryBusSelectName_2/9 -> __UniqueOutportName__13__/1  "<beta>"
  temporaryBusSelectName_2/8 -> __UniqueOutportName__12__/1  "<psi>"
  temporaryBusSelectName_2/7 -> __UniqueOutportName__11__/1  "<pos_y>"
  temporaryBusSelectName_2/6 -> __UniqueOutportName__10__/1  "<pos_x>"
  temporaryBusSelectName_2/5 -> __UniqueOutportName__9__/1  "<delta_v>"
  temporaryBusSelectName_2/4 -> __UniqueOutportName__8__/1  "<Fyh>"
  temporaryBusSelectName_2/3 -> __UniqueOutportName__7__/1  "<Fyv>"
  temporaryBusSelectName_2/2 -> __UniqueOutportName__6__/1  "<Fxh>"
  temporaryBusSelectName_2/1 -> __UniqueOutportName__5__/1  "<Fxv>"
  temporaryBusSelectName_1/4 -> __UniqueOutportName__4__/1  "<delta_v>"
  temporaryBusSelectName_1/3 -> __UniqueOutportName__3__/1  "<M_brems_h>"
  temporaryBusSelectName_1/2 -> __UniqueOutportName__2__/1  "<M_brems_v>"
  temporaryBusSelectName_1/1 -> __UniqueOutportName__1__/1  "<M_rad>"
  info_in/1 -> temporaryBusSelectName_3/1
  body dynamics/1 -> temporaryBusSelectName_2/1
  antrieb_in/1 -> temporaryBusSelectName_1/1

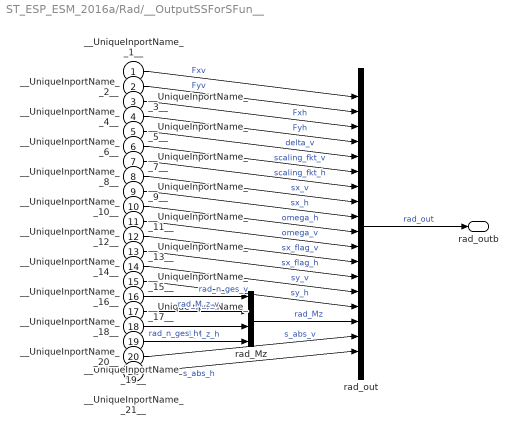
== system ST_ESP_ESM_2016a/Rad/__OutputSSForSFun__ ==
  __UniqueInportName__1__ : Inport
  __UniqueInportName__2__ : Inport  Port=2
  __UniqueInportName__3__ : Inport  Port=3
  __UniqueInportName__4__ : Inport  Port=4
  __UniqueInportName__5__ : Inport  Port=5
  __UniqueInportName__6__ : Inport  Port=6
  __UniqueInportName__7__ : Inport  Port=7
  __UniqueInportName__8__ : Inport  Port=8
  __UniqueInportName__9__ : Inport  Port=9
  __UniqueInportName__10__ : Inport  Port=10
  __UniqueInportName__11__ : Inport  Port=11
  __UniqueInportName__12__ : Inport  Port=12
  __UniqueInportName__13__ : Inport  Port=13
  __UniqueInportName__14__ : Inport  Port=14
  __UniqueInportName__15__ : Inport  Port=15
  __UniqueInportName__16__ : Inport  Port=16
  __UniqueInportName__17__ : Inport  Port=17
  __UniqueInportName__18__ : Inport  Port=18
  __UniqueInportName__19__ : Inport  Port=19
  __UniqueInportName__20__ : Inport  Port=20
  __UniqueInportName__21__ : Inport  Port=21
  rad_Mz : BusCreator  Inputs=4
  rad_out : BusCreator  Inputs=18
  rad_outb : Outport
  wires:
  rad_out/1 -> rad_outb/1  "rad_out"
  __UniqueInportName__21__/1 -> rad_out/18  "s_abs_h"
  __UniqueInportName__20__/1 -> rad_out/17  "s_abs_v"
  rad_Mz/1 -> rad_out/16  "rad_Mz"
  __UniqueInportName__15__/1 -> rad_out/15  "sy_h"
  __UniqueInportName__14__/1 -> rad_out/14  "sy_v"
  __UniqueInportName__13__/1 -> rad_out/13  "sx_flag_h"
  __UniqueInportName__12__/1 -> rad_out/12  "sx_flag_v"
  __UniqueInportName__11__/1 -> rad_out/11  "omega_v"
  __UniqueInportName__10__/1 -> rad_out/10  "omega_h"
  __UniqueInportName__9__/1 -> rad_out/9  "sx_h"
  __UniqueInportName__8__/1 -> rad_out/8  "sx_v"
  __UniqueInportName__7__/1 -> rad_out/7  "scaling_fkt_h"
  __UniqueInportName__6__/1 -> rad_out/6  "scaling_fkt_v"
  __UniqueInportName__5__/1 -> rad_out/5  "delta_v"
  __UniqueInportName__4__/1 -> rad_out/4  "Fyh"
  __UniqueInportName__3__/1 -> rad_out/3  "Fxh"
  __UniqueInportName__2__/1 -> rad_out/2  "Fyv"
  __UniqueInportName__1__/1 -> rad_out/1  "Fxv"
  __UniqueInportName__19__/1 -> rad_Mz/4  "rad_M_z_h"
  __UniqueInportName__18__/1 -> rad_Mz/3  "rad_n_ges_h"
  __UniqueInportName__17__/1 -> rad_Mz/2  "rad_M_z_v"
  __UniqueInportName__16__/1 -> rad_Mz/1  "rad_n_ges_v"

== system ST_ESP_ESM_2016a/Regelsysteme/ESP ==
  body dynamics : Inport
  Rad : Inport  Port=2
  umwelt : Inport  Port=3
  fah : Inport  Port=4
  Bus Selector2 : BusSelector  OutputSignals=rad_mue.rad_mue_vl,rad_mue.rad_mue_hl
  Bus Selector3 : BusSelector  OutputSignals=delta_v
  Bus Selector4 : BusSelector  OutputSignals=Fzv,Fzh,v,psi_p,beta
  Constant1 : Constant
  Constant3 : Constant  Value=0
  Filter : Subsystem
  PID-Regler : Subsystem
  Sensorik : Subsystem
  Soll_Gierrate : Subsystem
  c_alpha : Subsystem
      mask help: Simulink:masks:GenSFuncDesc_MD
      mask Help: eval('feval(''rtwprivate'',''rtwhelpview'',''rtw_sfcn_block'')');
  delta_Mz : Outport
  ESP_dkv : Outport  Port=2
  flag_beta_corr : Outport  Port=3
  psi_p_soll : Outport  Port=4
  wires:
  umwelt/1 -> Bus Selector2/1
  body dynamics/1 -> Bus Selector4/1
  Bus Selector4/3 -> Sensorik/1(v)  "<v>"
  Bus Selector4/4 -> Sensorik/2(psi_p)  "<psi_p>"
  Bus Selector4/5 -> Sensorik/3(beta)  "<beta>"
  Sensorik/1(v_mess) -> Filter/1(v_mess)
  Sensorik/2(psi_p_mess) -> Filter/2(psi_p_mess)
  Sensorik/3(beta_mess) -> Filter/3(beta_mess)
  Constant1/1 -> ESP_dkv/1
  fah/1 -> Bus Selector3/1
  Constant3/1 -> flag_beta_corr/1
  Soll_Gierrate/1("Soll_Gierrate ") -> PID-Regler/1(psi_p_soll), psi_p_soll/1
  Filter/1(v_filter) -> Soll_Gierrate/3(v_filter), PID-Regler/2(v_filter)
  Filter/2(psi_p_filter) -> PID-Regler/4(psi_p_filter)
  Filter/3(beta_filter) -> Soll_Gierrate/5(beta_filter), PID-Regler/3(beta_filter)
  Bus Selector2/1 -> c_alpha/1(mue_v)  "<rad_mue_vl>"
  Bus Selector2/2 -> c_alpha/2(mue_h)  "<rad_mue_hl>"
  Rad/1 -> c_alpha/3(Rad)
  Bus Selector4/1 -> c_alpha/4(Fzv)  "<Fzv>"
  Bus Selector4/2 -> c_alpha/5(Fzh)  "<Fzh>"
  Bus Selector3/1 -> Soll_Gierrate/4(delta_v)  "<delta_v>"
  c_alpha/1(c_alpha_v) -> Soll_Gierrate/1(c_alph_v)
  c_alpha/2(c_alpha_h) -> Soll_Gierrate/2(c_alph_h)
  PID-Regler/1(delta_Mz) -> delta_Mz/1

== system ST_ESP_ESM_2016a/Umwelt Info/mue_konst ==
  Bus Creator : BusCreator  Inputs=2
  Reibwert h : Constant  Value=mue_h
  Reibwert v : Constant  Value=mue_v
  rad_mue : Outport
  wires:
  Reibwert v/1 -> Bus Creator/1  "rad_mue_vl"
  Reibwert h/1 -> Bus Creator/2  "rad_mue_hl"
  Bus Creator/1 -> rad_mue/1  "rad_mue"

== system ST_ESP_ESM_2016a/Fahrzeug/Bewegungsgleichungen /a_x// a_y ==
  psi_p : Inport
  beta : Inport  Port=2
  beta_p : Inport  Port=3
  v_p : Inport  Port=4
  v : Inport  Port=5
  Add : Sum
  Add1 : Sum  Inputs=-+
  Add2 : Sum
  Product{,1..4} (5 alike) : Product
  Trigonometric Function : Trigonometry  Operator=cos
  Trigonometric Function3 : Trigonometry
  a_y : Outport
  a_x : Outport  Port=2
  wires:
  psi_p/1 -> Add/1
  beta_p/1 -> Add/2
  Add/1 -> Product/2
  v/1 -> Product/1
  beta/1 -> Trigonometric Function3/1, Trigonometric Function/1
  v_p/1 -> Product2/2, Product1/2
  Trigonometric Function/1 -> Product4/2, Product1/1
  Trigonometric Function3/1 -> Product2/1, Product3/2
  Product/1 -> Product3/1, Product4/1
  Product2/1 -> Add2/2
  Product4/1 -> Add2/1
  Product3/1 -> Add1/1
  Product1/1 -> Add1/2
  Add1/1 -> a_x/1
  Add2/1 -> a_y/1

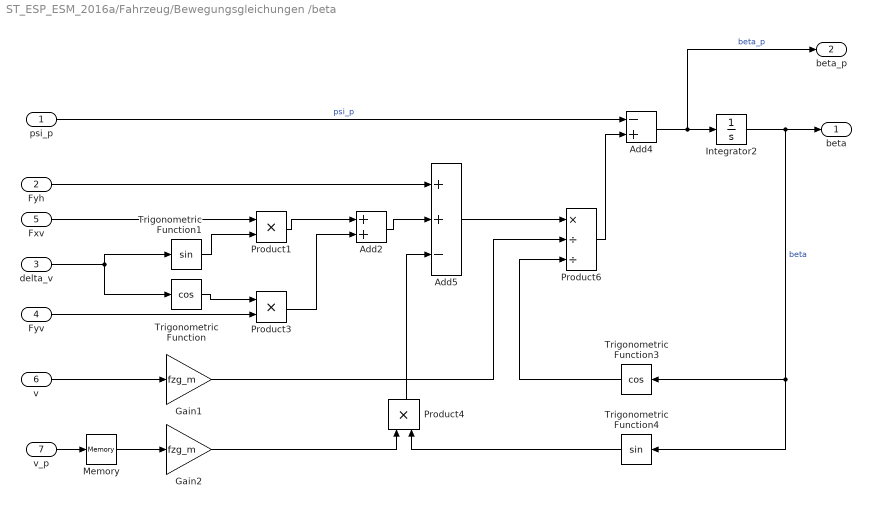
== system ST_ESP_ESM_2016a/Fahrzeug/Bewegungsgleichungen /beta  ==
  psi_p : Inport
  Fyh : Inport  Port=2
  delta_v : Inport  Port=3
  Fyv : Inport  Port=4
  Fxv : Inport  Port=5
  v : Inport  Port=6
  v_p : Inport  Port=7
  Add2 : Sum
  Add4 : Sum  Inputs=-+
  Add5 : Sum  Inputs=++-
  Gain1 : Gain  Gain=fzg_m
  Gain2 : Gain  Gain=fzg_m
  Integrator2 : Integrator
  Memory : Memory
  Product1 : Product
  Product3 : Product
  Product4 : Product
  Product6 : Product  Inputs=*//
  Trigonometric Function : Trigonometry  Operator=cos
  Trigonometric Function1 : Trigonometry
  Trigonometric Function3 : Trigonometry  Operator=cos
  Trigonometric Function4 : Trigonometry
  beta : Outport
  beta_p : Outport  Port=2
  wires:
  Integrator2/1 -> Trigonometric Function4/1, Trigonometric Function3/1, beta/1  "beta"
  psi_p/1 -> Add4/1  "psi_p"
  Add4/1 -> beta_p/1, Integrator2/1  "beta_p"
  Trigonometric Function3/1 -> Product6/3
  Product6/1 -> Add4/2
  v/1 -> Gain1/1
  Gain1/1 -> Product6/2
  Add5/1 -> Product6/1
  delta_v/1 -> Trigonometric Function/1, Trigonometric Function1/1
  Trigonometric Function1/1 -> Product1/2
  Product1/1 -> Add2/1
  Product3/1 -> Add2/2
  Fxv/1 -> Product1/1
  Trigonometric Function/1 -> Product3/1
  Fyv/1 -> Product3/2
  Fyh/1 -> Add5/1
  Add2/1 -> Add5/2
  v_p/1 -> Memory/1
  Gain2/1 -> Product4/1
  Trigonometric Function4/1 -> Product4/2
  Product4/1 -> Add5/3
  Memory/1 -> Gain2/1

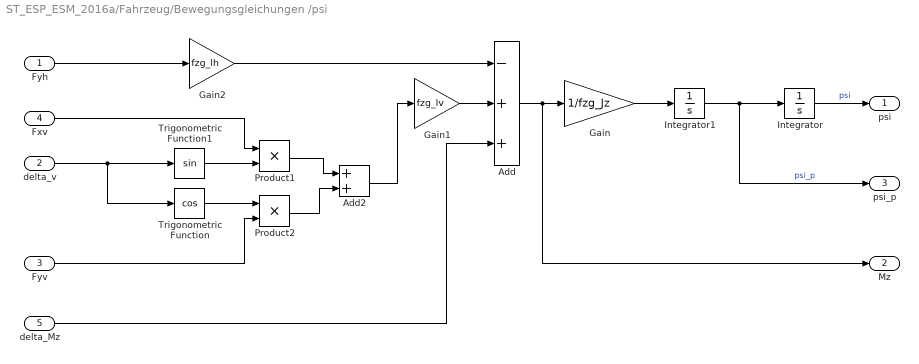
== system ST_ESP_ESM_2016a/Fahrzeug/Bewegungsgleichungen /psi  ==
  Fyh : Inport
  delta_v : Inport  Port=2
  Fyv : Inport  Port=3
  Fxv : Inport  Port=4
  delta_Mz : Inport  Port=5
  Add : Sum  Inputs=-++
  Add2 : Sum
  Gain : Gain  Gain=1/fzg_Jz
  Gain1 : Gain  Gain=fzg_lv
  Gain2 : Gain  Gain=fzg_lh
  Integrator : Integrator
  Integrator1 : Integrator
  Product1 : Product
  Product2 : Product
  Trigonometric Function : Trigonometry  Operator=cos
  Trigonometric Function1 : Trigonometry
  psi : Outport
  Mz : Outport  Port=2
  psi_p : Outport  Port=3
  wires:
  Integrator1/1 -> Integrator/1, psi_p/1  "psi_p"
  Integrator/1 -> psi/1  "psi"
  Gain/1 -> Integrator1/1
  Add/1 -> Gain/1, Mz/1
  Gain2/1 -> Add/1
  Fyh/1 -> Gain2/1
  delta_v/1 -> Trigonometric Function/1, Trigonometric Function1/1
  Trigonometric Function1/1 -> Product1/2
  Product1/1 -> Add2/1
  Product2/1 -> Add2/2
  Fxv/1 -> Product1/1
  Trigonometric Function/1 -> Product2/1
  Fyv/1 -> Product2/2
  Add2/1 -> Gain1/1
  Gain1/1 -> Add/2
  delta_Mz/1 -> Add/3

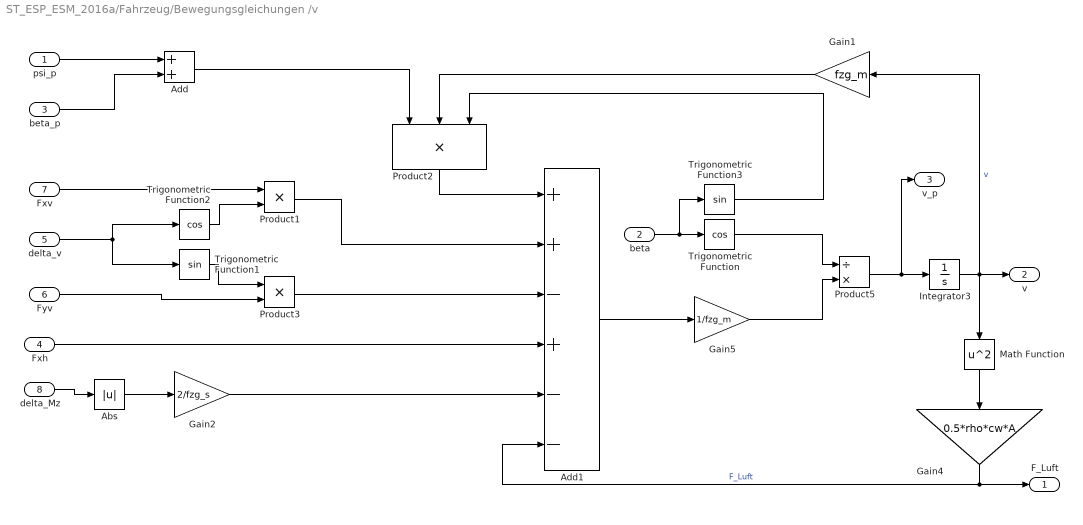
== system ST_ESP_ESM_2016a/Fahrzeug/Bewegungsgleichungen /v  ==
  psi_p : Inport
  beta : Inport  Port=2
  beta_p : Inport  Port=3
  Fxh : Inport  Port=4
  delta_v : Inport  Port=5
  Fyv : Inport  Port=6
  Fxv : Inport  Port=7
  delta_Mz : Inport  Port=8
  Abs : Abs
  Add : Sum
  Add1 : Sum  Inputs=++-+--
  Gain1 : Gain  Gain=fzg_m
  Gain2 : Gain  Gain=2/fzg_s
  Gain4 : Gain  Gain=0.5*rho*cw*A
  Gain5 : Gain  Gain=1/fzg_m
  Integrator3 : Integrator  InitialCondition=init_v0
  Math Function : Math  Operator=square  SaturateOnIntegerOverflow=on
  Product1 : Product
  Product2 : Product  Inputs=3
  Product3 : Product
  Product5 : Product  Inputs=/*
  Trigonometric Function : Trigonometry  Operator=cos
  Trigonometric Function1 : Trigonometry
  Trigonometric Function2 : Trigonometry  Operator=cos
  Trigonometric Function3 : Trigonometry
  F_Luft : Outport
  v : Outport  Port=2
  v_p : Outport  Port=3
  wires:
  Integrator3/1 -> v/1, Gain1/1, Math Function/1  "v"
  Gain4/1 -> F_Luft/1, Add1/6  "F_Luft"
  Math Function/1 -> Gain4/1
  Product2/1 -> Add1/1
  Fxh/1 -> Add1/4
  Product3/1 -> Add1/3
  Product1/1 -> Add1/2
  Add1/1 -> Gain5/1
  Gain5/1 -> Product5/2
  beta/1 -> Trigonometric Function3/1, Trigonometric Function/1
  Product5/1 -> v_p/1, Integrator3/1
  delta_v/1 -> Trigonometric Function2/1, Trigonometric Function1/1
  Trigonometric Function2/1 -> Product1/2
  Fxv/1 -> Product1/1
  Trigonometric Function1/1 -> Product3/1
  Fyv/1 -> Product3/2
  psi_p/1 -> Add/1
  beta_p/1 -> Add/2
  Trigonometric Function/1 -> Product5/1
  Trigonometric Function3/1 -> Product2/3
  Gain1/1 -> Product2/2
  Add/1 -> Product2/1
  delta_Mz/1 -> Abs/1
  Gain2/1 -> Add1/5
  Abs/1 -> Gain2/1

== system ST_ESP_ESM_2016a/Regelsysteme/ESP/Filter ==
  v_mess : Inport
  psi_p_mess : Inport  Port=2
  beta_mess : Inport  Port=3
  To Workspace : ToWorkspace  VariableName=v_mess  SampleTime=-1
  To Workspace1 : ToWorkspace  VariableName=psi_p_mess  SampleTime=-1
  To Workspace2 : ToWorkspace  VariableName=beta_mess  SampleTime=-1
  To Workspace3 : ToWorkspace  VariableName=v_filter  SampleTime=-1
  To Workspace4 : ToWorkspace  VariableName=psi_p_filter  SampleTime=-1
  To Workspace5 : ToWorkspace  VariableName=beta_filter  SampleTime=-1
  Transfer Fcn : TransferFcn  Denominator=[0.0125 1]
  Transfer Fcn1 : TransferFcn  Denominator=[0.025 1]
  Transfer Fcn2 : TransferFcn  Denominator=[0.125 1]
  v_filter : Outport
  psi_p_filter : Outport  Port=2
  beta_filter : Outport  Port=3
  wires:
  v_mess/1 -> To Workspace/1, Transfer Fcn/1
  psi_p_mess/1 -> To Workspace1/1, Transfer Fcn1/1
  beta_mess/1 -> To Workspace2/1, Transfer Fcn2/1
  Transfer Fcn/1 -> To Workspace3/1, v_filter/1
  Transfer Fcn1/1 -> To Workspace4/1, psi_p_filter/1
  Transfer Fcn2/1 -> To Workspace5/1, beta_filter/1

== system ST_ESP_ESM_2016a/Regelsysteme/ESP/PID-Regler ==
  psi_p_soll : Inport
  v_filter : Inport  Port=2
  beta_filter : Inport  Port=3
  psi_p_filter : Inport  Port=4
  Abs1 : Abs
  D-Anteil : MATLAB Function  TreatAsAtomicUnit=on
      settings: PermitHierarchicalResolution=ParametersOnly
  Dead Zone : MATLAB Function  TreatAsAtomicUnit=on
      settings: PermitHierarchicalResolution=ParametersOnly
  Derivative : Derivative
  I-Anteil : MATLAB Function  TreatAsAtomicUnit=on
      settings: PermitHierarchicalResolution=ParametersOnly
  Integrator : Integrator  ExternalReset=level
  Memory : Memory
  P-Anteil : MATLAB Function  TreatAsAtomicUnit=on
      settings: PermitHierarchicalResolution=ParametersOnly
  Sum : Sum  Inputs=+++
  Sum1 : Sum  Inputs=|+-
  Sum2 : Sum  Inputs=|+-
  delta_Mz : Outport
  wires:
  Memory/1 -> Abs1/1
  Sum/1 -> Sum1/1, Dead Zone/1(u)  "delta_Mz"
  P-Anteil/1(y) -> Sum/1
  I-Anteil/1(y) -> Sum/3
  Dead Zone/1(y) -> delta_Mz/1, Sum1/2
  Integrator/1 -> I-Anteil/1(psi_p)
  Sum2/1 -> Integrator/1, Derivative/1, P-Anteil/1(psi_p)
  Derivative/1 -> D-Anteil/1(psi_p)
  D-Anteil/1(y) -> Sum/2
  Sum1/1 -> Memory/1
  v_filter/1 -> I-Anteil/2(v), D-Anteil/2(v), P-Anteil/3(v)
  Abs1/1 -> Integrator/2
  psi_p_filter/1 -> Sum2/2
  beta_filter/1 -> P-Anteil/2(beta)
  psi_p_soll/1 -> Sum2/1

== system ST_ESP_ESM_2016a/Regelsysteme/ESP/Sensorik ==
  v : Inport
  psi_p : Inport  Port=2
  beta : Inport  Port=3
  Geschwindigkeitssensor : Subsystem
  Gierratensensor : Subsystem
  Schwimmwinkelsensor : Subsystem
  v_mess : Outport
  psi_p_mess : Outport  Port=2
  beta_mess : Outport  Port=3
  wires:
  Geschwindigkeitssensor/1(v_mess) -> v_mess/1
  psi_p/1 -> Gierratensensor/1(psi_p)
  beta/1 -> Schwimmwinkelsensor/1(beta)
  Gierratensensor/1(psi_p_mess) -> psi_p_mess/1
  Schwimmwinkelsensor/1(beta_mess) -> beta_mess/1
  v/1 -> Geschwindigkeitssensor/1(v)

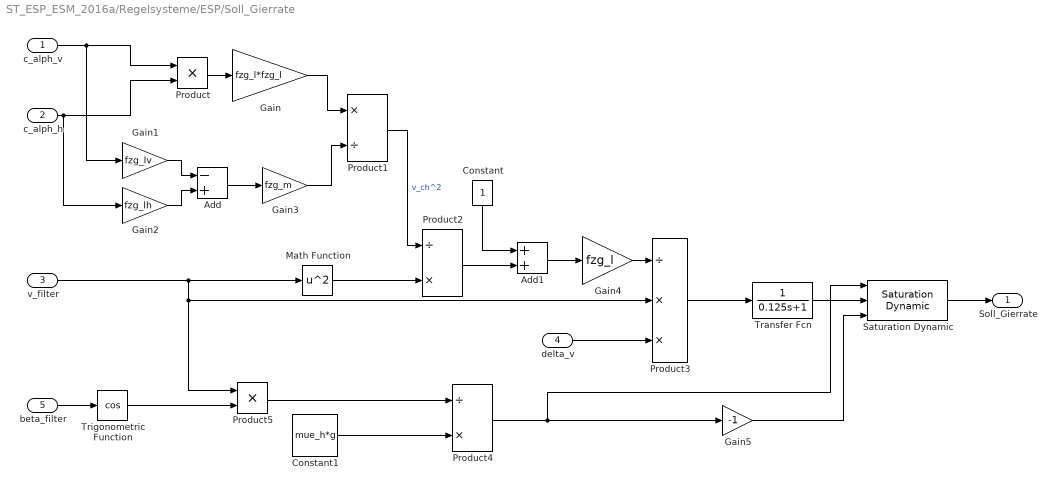
== system ST_ESP_ESM_2016a/Regelsysteme/ESP/Soll_Gierrate ==
  c_alph_v : Inport
  c_alph_h : Inport  Port=2
  v_filter : Inport  Port=3
  delta_v : Inport  Port=4
  beta_filter : Inport  Port=5
  Add : Sum  Inputs=-+
  Add1 : Sum
  Constant : Constant  VectorParams1D=off  SampleTime=-1
  Constant1 : Constant  Value=mue_h*g
  Gain : Gain  Gain=fzg_l*fzg_l
  Gain1 : Gain  Gain=fzg_lv
  Gain2 : Gain  Gain=fzg_lh
  Gain3 : Gain  Gain=fzg_m
  Gain4 : Gain  Gain=fzg_l
  Gain5 : Gain  Gain=-1
  Math Function : Math  Operator=square  SaturateOnIntegerOverflow=on
  Product : Product
  Product1 : Product  Inputs=*/
  Product2 : Product  Inputs=/*
  Product3 : Product  Inputs=/**
  Product4 : Product  Inputs=/*
  Product5 : Product
  Saturation Dynamic : simulink/Discontinuities/Saturation Dynamic  OutMin=[]  OutMax=[]  OutDataTypeStr=Inherit: Same as second input  OutDataType=fixdt(1, 16)  OutScaling=2^-10  DoSatur=off
  Transfer Fcn : TransferFcn  Denominator=[0.125 1]
  Trigonometric Function : Trigonometry  Operator=cos
  "Soll_Gierrate " : Outport
  wires:
  c_alph_h/1 -> Gain2/1, Product/2
  Product/1 -> Gain/1
  c_alph_v/1 -> Gain1/1, Product/1
  Gain1/1 -> Add/1
  Gain2/1 -> Add/2
  Add/1 -> Gain3/1
  Gain/1 -> Product1/1
  Gain3/1 -> Product1/2
  v_filter/1 -> Product5/1, Product3/2, Math Function/1
  Math Function/1 -> Product2/2
  Product1/1 -> Product2/1  "v_ch^2"
  Product2/1 -> Add1/2
  Constant/1 -> Add1/1
  Add1/1 -> Gain4/1
  Gain4/1 -> Product3/1
  delta_v/1 -> Product3/3
  Product3/1 -> Transfer Fcn/1
  Constant1/1 -> Product4/2
  Product4/1 -> Saturation Dynamic/1, Gain5/1
  Transfer Fcn/1 -> Saturation Dynamic/2
  Saturation Dynamic/1 -> "Soll_Gierrate "/1
  Gain5/1 -> Saturation Dynamic/3
  Product5/1 -> Product4/1
  beta_filter/1 -> Trigonometric Function/1
  Trigonometric Function/1 -> Product5/2

== system ST_ESP_ESM_2016a/Regelsysteme/ESP/c_alpha ==
  mue_v : Inport
  mue_h : Inport  Port=2
  Rad : Inport  Port=3
  Fzv : Inport  Port=4
  Fzh : Inport  Port=5
  __InputSSForSFun__ : Subsystem
      settings: PermitHierarchicalResolution=ParametersOnly
  __OutputSSForSFun__ : Subsystem
      settings: PermitHierarchicalResolution=ParametersOnly
  c_alpha_sfcn : S-Function  FunctionName=c_alpha_sf  SFunctionModules=""  SFunctionDeploymentMode=off  EnableBusSupport=off  mask{rtw_sf_name=c_alpha_sf, showVar=off}
      mask prompts: rtw_sf_name "Simulink:masks:GenSFuncName_MP"; showVar "Simulink:masks:GenSFuncShowModuleList_MP"
      mask help: Simulink:masks:GenSFuncDesc_MD
      mask init: same as ST_ESP_ESM_2016a/Rad/Rad_sfcn
      settings: CopyFcn=|
      | if ~strcmp(get_param(gcb,'Linkstatus'),'none') && ...
      | ~strcmp(get_param(gcb,'Linkstatus'),'implicit')
      |   set_param(gcb,'LinkStatus','none');
      | end
      mask Help: eval('feval(''rtwprivate'',''rtwhelpview'',''rtw_sfcn_block'')');
      mask Display:
      | port_label('input',1,'mue_v');
      | port_label('input',2,'mue_h');
      | port_label('input',3,'Fxv');
      | port_label('input',4,'Fyv');
      | port_label('input',5,'Fxh');
      | port_label('input',6,'Fyh');
      | port_label('input',7,'delta_v');
      | port_label('input',8,'scaling_fkt_v');
      | port_label('input',9,'scaling_fkt_h');
      | port_label('input',10,'sx_v');
      | port_label('input',11,'sx_h');
      | port_label('input',12,'omega_h');
      | port_label('input',13,'omega_v');
      | port_label('input',14,'sx_flag_v');
      | port_label('input',15,'sx_flag_h');
      | port_label('input',16,'sy_v');
      | port_label('input',17,'sy_h');
      | port_label('input',18,'rad_n_ges_v');
      | port_label('input',19,'rad_M_z_v');
      | port_label('input',20,'rad_n_ges_h');
      | port_label('input',21,'rad_M_z_h');
      | port_label('input',22,'s_abs_v');
      | port_label('input',23,'s_abs_h');
      | port_label('input',24,'Fzv');
      | port_label('input',25,'Fzh');
      | port_label('output',1,'c_alpha_v');
      | port_label('output',2,'c_alpha_h');
  c_alpha_v : Outport
  c_alpha_h : Outport  Port=2
  wires:
  __OutputSSForSFun__/2(c_alpha_h) -> c_alpha_h/1
  __OutputSSForSFun__/1(c_alpha_v) -> c_alpha_v/1
  c_alpha_sfcn/2 -> __OutputSSForSFun__/2(__UniqueInportName__2__)
  c_alpha_sfcn/1 -> __OutputSSForSFun__/1(__UniqueInportName__1__)
  __InputSSForSFun__/25(__UniqueOutportName__25__) -> c_alpha_sfcn/25
  __InputSSForSFun__/24(__UniqueOutportName__24__) -> c_alpha_sfcn/24
  __InputSSForSFun__/23(__UniqueOutportName__23__) -> c_alpha_sfcn/23
  __InputSSForSFun__/22(__UniqueOutportName__22__) -> c_alpha_sfcn/22
  __InputSSForSFun__/21(__UniqueOutportName__21__) -> c_alpha_sfcn/21
  __InputSSForSFun__/20(__UniqueOutportName__20__) -> c_alpha_sfcn/20
  __InputSSForSFun__/19(__UniqueOutportName__19__) -> c_alpha_sfcn/19
  __InputSSForSFun__/18(__UniqueOutportName__18__) -> c_alpha_sfcn/18
  __InputSSForSFun__/17(__UniqueOutportName__17__) -> c_alpha_sfcn/17
  __InputSSForSFun__/16(__UniqueOutportName__16__) -> c_alpha_sfcn/16
  __InputSSForSFun__/15(__UniqueOutportName__15__) -> c_alpha_sfcn/15
  __InputSSForSFun__/14(__UniqueOutportName__14__) -> c_alpha_sfcn/14
  __InputSSForSFun__/13(__UniqueOutportName__13__) -> c_alpha_sfcn/13
  __InputSSForSFun__/12(__UniqueOutportName__12__) -> c_alpha_sfcn/12
  __InputSSForSFun__/11(__UniqueOutportName__11__) -> c_alpha_sfcn/11
  __InputSSForSFun__/10(__UniqueOutportName__10__) -> c_alpha_sfcn/10
  __InputSSForSFun__/9(__UniqueOutportName__9__) -> c_alpha_sfcn/9
  __InputSSForSFun__/8(__UniqueOutportName__8__) -> c_alpha_sfcn/8
  __InputSSForSFun__/7(__UniqueOutportName__7__) -> c_alpha_sfcn/7
  __InputSSForSFun__/6(__UniqueOutportName__6__) -> c_alpha_sfcn/6
  __InputSSForSFun__/5(__UniqueOutportName__5__) -> c_alpha_sfcn/5
  __InputSSForSFun__/4(__UniqueOutportName__4__) -> c_alpha_sfcn/4
  __InputSSForSFun__/3(__UniqueOutportName__3__) -> c_alpha_sfcn/3
  __InputSSForSFun__/2(__UniqueOutportName__2__) -> c_alpha_sfcn/2
  __InputSSForSFun__/1(__UniqueOutportName__1__) -> c_alpha_sfcn/1
  Fzh/1 -> __InputSSForSFun__/5(Fzh)
  Fzv/1 -> __InputSSForSFun__/4(Fzv)
  Rad/1 -> __InputSSForSFun__/3(Rad)
  mue_h/1 -> __InputSSForSFun__/2(mue_h)
  mue_v/1 -> __InputSSForSFun__/1(mue_v)

== system ST_ESP_ESM_2016a/Regelsysteme/ESP/Sensorik/Geschwindigkeitssensor ==
  v : Inport
  Offset : Constant  Value=0.01
  Product : Product  RndMeth=Zero
  Rate Transition : RateTransition
  Rauschamplitude : Constant  Value=0.01
  Sum : Sum  Inputs=+++
  Uniform Random Number : UniformRandomNumber  SampleTime=0.1
  v_mess : Outport
  wires:
  v/1 -> Sum/1
  Product/1 -> Sum/2
  Rauschamplitude/1 -> Product/1
  Rate Transition/1 -> Product/2
  Offset/1 -> Sum/3
  Sum/1 -> v_mess/1
  Uniform Random Number/1 -> Rate Transition/1

== system ST_ESP_ESM_2016a/Regelsysteme/ESP/Sensorik/Gierratensensor ==
  psi_p : Inport
  Offset : Constant  Value=0.01
  Product : Product  RndMeth=Zero
  Rate Transition : RateTransition
  Rauschamplitude : Constant  Value=0.004
  Sum : Sum  Inputs=+++
  Uniform Random Number : UniformRandomNumber  SampleTime=0.1
  psi_p_mess : Outport
  wires:
  psi_p/1 -> Sum/1
  Product/1 -> Sum/2
  Rauschamplitude/1 -> Product/1
  Rate Transition/1 -> Product/2
  Offset/1 -> Sum/3
  Sum/1 -> psi_p_mess/1
  Uniform Random Number/1 -> Rate Transition/1
